simulink model "Implicative_2"  (R2016a)
settings: Solver=VariableStepAuto  StartTime=0.0  StopTime=15  RelTol=1e-3
values from neighbouring files (symbols this model uses):
  A = [ ... (first row only)    [Implicative_Model.m]
  B = [ ... (first row only)    [Implicative_Model.m]
  B_inv = inv(B'*B)*B'    [Implicative_Model.m]
  collective = 0    [Implicative_Model.m]
  H2 = inv(B'*B)*B'*B2d    [Implicative_Model.m]
  K2 = inv((B'*B))*B'*(A-A2d)    [Implicative_Model.m]
  lateral = 0    [Implicative_Model.m]
  longtudinal = 1    [Implicative_Model.m]
  pedal = 0    [Implicative_Model.m]
settings Model: Creator=Administrator  LastModifiedBy=Administrator

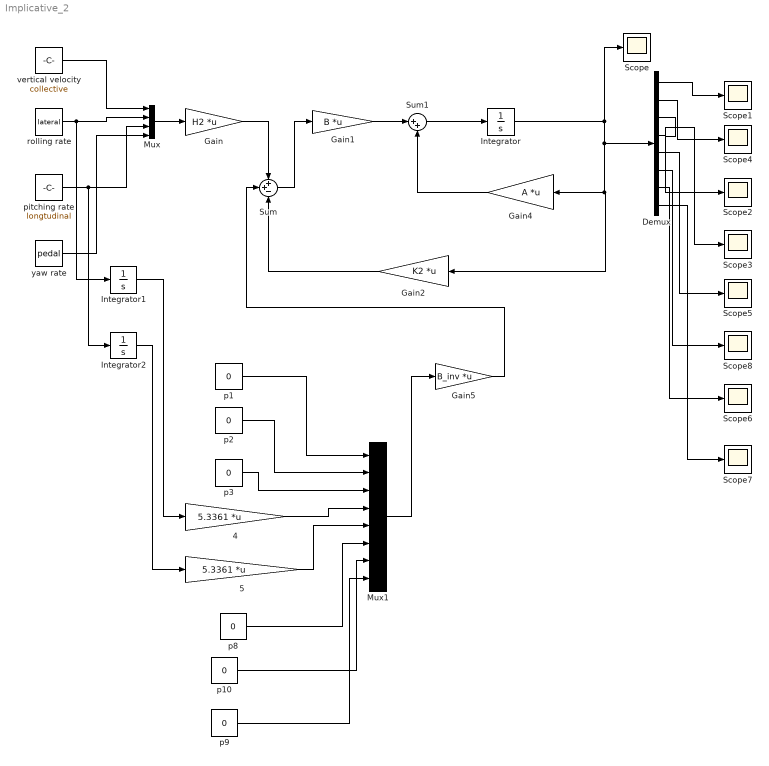
== system Implicative_2 ==
  4 : Gain  Gain=5.3361  Multiplication=Matrix(K*u)
  5 : Gain  Gain=5.3361  Multiplication=Matrix(K*u)
  Demux : Demux  Outputs=8
  Gain : Gain  Gain=H2  Multiplication=Matrix(K*u)
  Gain1 : Gain  Gain=B  Multiplication=Matrix(K*u)
  Gain2 : Gain  Gain=K2  Multiplication=Matrix(K*u)
  Gain4 : Gain  Gain=A  Multiplication=Matrix(K*u)
  Gain5 : Gain  Gain=B_inv  Multiplication=Matrix(K*u)
  Integrator : Integrator
  Integrator1 : Integrator
  Integrator2 : Integrator
  Mux : Mux
  Mux1 : Mux  Inputs=8
  Scope{,1..8} (9 alike) : Scope
  Sum : Sum  Inputs=++-
  Sum1 : Sum  Inputs=|++
  p{1..3,8..10} (6 alike) : Constant  Value=0
  pitching rate : Constant  Value=longtudinal
  rolling rate : Constant  Value=lateral
  vertical velocity : Constant  Value=collective
  yaw rate : Constant  Value=pedal
  wires:
  vertical velocity/1 -> Mux/1
  rolling rate/1 -> Integrator1/1, Mux/2
  pitching rate/1 -> Integrator2/1, Mux/3
  yaw rate/1 -> Mux/4
  Mux/1 -> Gain/1
  Sum/1 -> Gain1/1
  Sum1/1 -> Integrator/1
  Integrator/1 -> Demux/1, Gain2/1, Gain4/1, Scope/1
  Gain4/1 -> Sum1/2
  Gain1/1 -> Sum1/1
  Demux/1 -> Scope1/1
  Demux/2 -> Scope4/1
  Demux/3 -> Scope2/1
  Demux/4 -> Scope3/1
  Demux/5 -> Scope5/1
  Demux/6 -> Scope8/1
  Demux/7 -> Scope6/1
  Demux/8 -> Scope7/1
  Gain/1 -> Sum/1
  Gain2/1 -> Sum/3
  Gain5/1 -> Sum/2
  Mux1/1 -> Gain5/1
  p1/1 -> Mux1/1
  p2/1 -> Mux1/2
  p3/1 -> Mux1/3
  4/1 -> Mux1/4
  5/1 -> Mux1/5
  p8/1 -> Mux1/6
  p10/1 -> Mux1/7
  p9/1 -> Mux1/8
  Integrator1/1 -> 4/1
  Integrator2/1 -> 5/1
